simulink library "csc_src_slant_range_covariance_lib"  (R2015b)
settings: Solver=VariableStepAuto  StartTime=0.0  StopTime=10.0  RelTol=1e-3
values from neighbouring files (symbols this model uses):
  mnc_dtheta_filter_coeffs = [fir1(mnc_dtheta_filter_order(1),mnc_dtheta_filter_freq(1));,                               fir1(mnc_dtheta_filter_order(2),mnc_dtheta_filter_freq(2))]    [csc_mnc_measurement_noise_covariance_init.m]
  mnc_dtheta_filter_order = [1      1]    [csc_mnc_measurement_noise_covariance_init.m]
  mnc_meas_noise_alt = 8000.0    (= 8000)    [csc_mnc_measurement_noise_covariance_init.m]
  mnc_meas_noise_alt_gain = [0.2    0.2     1000   1000]    [csc_mnc_measurement_noise_covariance_init.m]
  mnc_meas_noise_angle_exp = [10     10]    [csc_mnc_measurement_noise_covariance_init.m]
  mnc_meas_noise_angle_gain = [1.0    1.0]    [csc_mnc_measurement_noise_covariance_init.m]
  mnc_meas_noise_angle_high = [90.0   20.0]    [csc_mnc_measurement_noise_covariance_init.m]
  mnc_meas_noise_angle_low = [10.0   10.0]    [csc_mnc_measurement_noise_covariance_init.m]
  mnc_meas_noise_angle_terminal = [10.0   10.0]    [csc_mnc_measurement_noise_covariance_init.m]
  mnc_meas_noise_dtheta = [4.0    4.0]    [csc_mnc_measurement_noise_covariance_init.m]
  mnc_meas_noise_dtheta_exp = [11     11]    [csc_mnc_measurement_noise_covariance_init.m]
  mnc_meas_noise_dtheta_gain = [0.0    0.0]    [csc_mnc_measurement_noise_covariance_init.m]
  mnc_nadir_cant_angle = [0.0   45.0]    [csc_mnc_measurement_noise_covariance_init.m]
  mnc_noise_switch_alt = [2000  2000]    [csc_mnc_measurement_noise_covariance_init.m]
  mnc_noise_terminal_alt = [ 100   100]    [csc_mnc_measurement_noise_covariance_init.m]
  mnc_R_lower_limit_alt = [0.0001 0.0001  10     10]    [csc_mnc_measurement_noise_covariance_init.m]
  mnc_R_lower_limit_angle = [0.0001 0.001]    [csc_mnc_measurement_noise_covariance_init.m]
  mnc_R_lower_limit_dtheta = [0.0001 0.0001]    [csc_mnc_measurement_noise_covariance_init.m]
libraries: simulink x8, util_info_lib x2
settings Model: Creator=Mark Agbayani  LastModifiedBy=Mark Agbayani

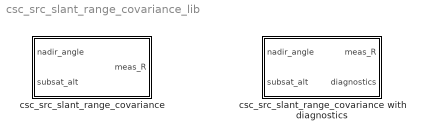
== system csc_src_slant_range_covariance_lib ==
  csc_src_slant_range_covariance : Subsystem  mask{i=0}
      mask prompts: i "Lidar Number"
  csc_src_slant_range_covariance with diagnostics : Subsystem  mask{i=0}
      mask prompts: i "Lidar Number"

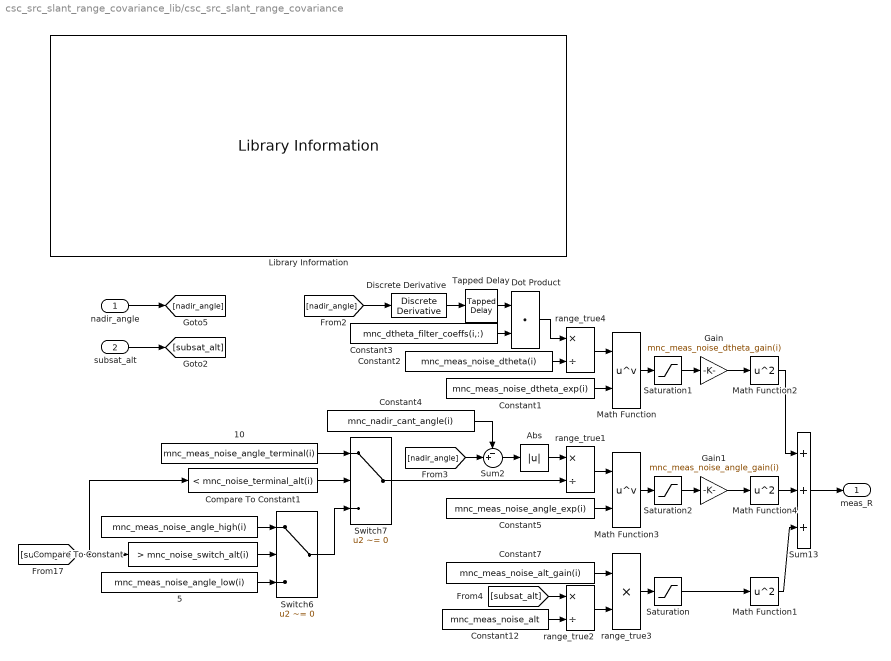
== system csc_src_slant_range_covariance_lib/csc_src_slant_range_covariance ==
  nadir_angle : Inport
  subsat_alt : Inport  Port=2
  "      " : Constant  Value=mnc_meas_noise_angle_high(i)
  "      10" : Constant  Value=mnc_meas_noise_angle_terminal(i)
  "      5" : Constant  Value=mnc_meas_noise_angle_low(i)
  Abs : Abs
  Compare To Constant : simulink/Logic and Bit Operations/Compare To Constant  relop=>  const=mnc_noise_switch_alt(i)  OutDataTypeStr=boolean
  Compare To Constant1 : simulink/Logic and Bit Operations/Compare To Constant  relop=<  const=mnc_noise_terminal_alt(i)  OutDataTypeStr=boolean
  Constant1 : Constant  Value=mnc_meas_noise_dtheta_exp(i)
  Constant12 : Constant  Value=mnc_meas_noise_alt
  Constant2 : Constant  Value=mnc_meas_noise_dtheta(i)
  Constant3 : Constant  Value=mnc_dtheta_filter_coeffs(i,:)
  Constant4 : Constant  Value=mnc_nadir_cant_angle(i)
  Constant5 : Constant  Value=mnc_meas_noise_angle_exp(i)
  Constant7 : Constant  Value=mnc_meas_noise_alt_gain(i)
  Discrete Derivative : simulink/Discrete/Discrete Derivative  gainval=1.0  ICPrevScaledInput=0.0  InputProcessing=Inherited  OutMin=[]  OutMax=[]  OutDataType=fixdt(1, 16)  OutScaling=2^-10  DoSatur=off
  Dot Product : DotProduct  InputSameDT=on  OutDataTypeStr=Inherit: Inherit via internal rule
  Gain : Gain  Gain=mnc_meas_noise_dtheta_gain(i)
  Gain1 : Gain  Gain=mnc_meas_noise_angle_gain(i)
  Library Information : util_info_lib/Library Information  owner='NONE'
  Math Function : Math  Operator=pow  SaturateOnIntegerOverflow=on
  Math Function1 : Math  Operator=square  SaturateOnIntegerOverflow=on
  Math Function2 : Math  Operator=square  SaturateOnIntegerOverflow=on
  Math Function3 : Math  Operator=pow  SaturateOnIntegerOverflow=on
  Math Function4 : Math  Operator=square  SaturateOnIntegerOverflow=on
  Saturation : Saturate  UpperLimit=1e20  LowerLimit=mnc_R_lower_limit_alt(i)
  Saturation1 : Saturate  UpperLimit=1e20  LowerLimit=mnc_R_lower_limit_dtheta(i)
  Saturation2 : Saturate  UpperLimit=1e20  LowerLimit=mnc_R_lower_limit_angle(i)
  Sum13 : Sum  Inputs=+++
  Sum2 : Sum  Inputs=-+|  AccumDataTypeStr=double
  Switch6 : Switch  Criteria=u2 ~= 0
  Switch7 : Switch  Criteria=u2 ~= 0
  Tapped Delay : simulink/Discrete/Tapped Delay  vinit=0.0  samptime=-1  NumDelays=mnc_dtheta_filter_order(i)  DelayOrder=Oldest  includeCurrent=on
  range_true1 : Product  Inputs=*/  RndMeth=Zero
  range_true2 : Product  Inputs=*/  RndMeth=Zero
  range_true3 : Product  RndMeth=Zero
  range_true4 : Product  Inputs=*/  RndMeth=Zero
  meas_R : Outport
  wires:
  nadir_angle/1 -> [nadir_angle]
  subsat_alt/1 -> [subsat_alt]
  Dot Product/1 -> range_true4/1
  Discrete Derivative/1 -> Tapped Delay/1
  Gain/1 -> Math Function2/1
  Gain1/1 -> Math Function4/1
  Constant5/1 -> Math Function3/2
  [nadir_angle] -> Discrete Derivative/1
  Switch7/1 -> range_true1/2
  Constant1/1 -> Math Function/2
  range_true1/1 -> Math Function3/1
  Math Function3/1 -> Saturation2/1
  Saturation2/1 -> Gain1/1
  Constant3/1 -> Dot Product/2
  Tapped Delay/1 -> Dot Product/1
  Math Function2/1 -> Sum13/1
  Constant2/1 -> range_true4/2
  range_true4/1 -> Math Function/1
  Math Function/1 -> Saturation1/1
  Saturation1/1 -> Gain/1
  Switch6/1 -> Switch7/3
  "      "/1 -> Switch6/1
  "      5"/1 -> Switch6/3
  Compare To Constant/1 -> Switch6/2
  [subsat_alt] -> Compare To Constant1/1, Compare To Constant/1
  "      10"/1 -> Switch7/1
  Compare To Constant1/1 -> Switch7/2
  Math Function4/1 -> Sum13/2
  range_true2/1 -> range_true3/2
  Constant7/1 -> range_true3/1
  range_true3/1 -> Saturation/1
  [subsat_alt] -> range_true2/1
  Constant12/1 -> range_true2/2
  Math Function1/1 -> Sum13/3
  Saturation/1 -> Math Function1/1
  Sum13/1 -> meas_R/1
  Constant4/1 -> Sum2/1
  Sum2/1 -> Abs/1
  [nadir_angle] -> Sum2/2
  Abs/1 -> range_true1/1

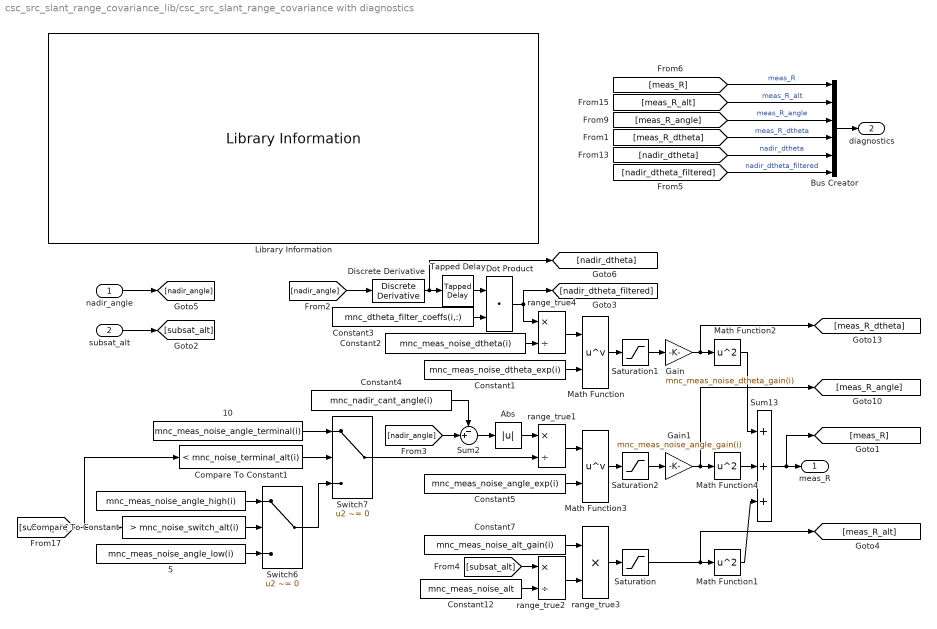
== system csc_src_slant_range_covariance_lib/csc_src_slant_range_covariance with diagnostics ==
  nadir_angle : Inport
  subsat_alt : Inport  Port=2
  "      " : Constant  Value=mnc_meas_noise_angle_high(i)
  "      10" : Constant  Value=mnc_meas_noise_angle_terminal(i)
  "      5" : Constant  Value=mnc_meas_noise_angle_low(i)
  Abs : Abs
  Bus Creator : BusCreator  Inputs=6
  Compare To Constant : simulink/Logic and Bit Operations/Compare To Constant  relop=>  const=mnc_noise_switch_alt(i)  OutDataTypeStr=boolean
  Compare To Constant1 : simulink/Logic and Bit Operations/Compare To Constant  relop=<  const=mnc_noise_terminal_alt(i)  OutDataTypeStr=boolean
  Constant1 : Constant  Value=mnc_meas_noise_dtheta_exp(i)
  Constant12 : Constant  Value=mnc_meas_noise_alt
  Constant2 : Constant  Value=mnc_meas_noise_dtheta(i)
  Constant3 : Constant  Value=mnc_dtheta_filter_coeffs(i,:)
  Constant4 : Constant  Value=mnc_nadir_cant_angle(i)
  Constant5 : Constant  Value=mnc_meas_noise_angle_exp(i)
  Constant7 : Constant  Value=mnc_meas_noise_alt_gain(i)
  Discrete Derivative : simulink/Discrete/Discrete Derivative  gainval=1.0  ICPrevScaledInput=0.0  InputProcessing=Inherited  OutMin=[]  OutMax=[]  OutDataType=fixdt(1, 16)  OutScaling=2^-10  DoSatur=off
  Dot Product : DotProduct  InputSameDT=on  OutDataTypeStr=Inherit: Inherit via internal rule
  Gain : Gain  Gain=mnc_meas_noise_dtheta_gain(i)
  Gain1 : Gain  Gain=mnc_meas_noise_angle_gain(i)
  Library Information : util_info_lib/Library Information  owner='NONE'
  Math Function : Math  Operator=pow  SaturateOnIntegerOverflow=on
  Math Function1 : Math  Operator=square  SaturateOnIntegerOverflow=on
  Math Function2 : Math  Operator=square  SaturateOnIntegerOverflow=on
  Math Function3 : Math  Operator=pow  SaturateOnIntegerOverflow=on
  Math Function4 : Math  Operator=square  SaturateOnIntegerOverflow=on
  Saturation : Saturate  UpperLimit=1e20  LowerLimit=mnc_R_lower_limit_alt(i)
  Saturation1 : Saturate  UpperLimit=1e20  LowerLimit=mnc_R_lower_limit_dtheta(i)
  Saturation2 : Saturate  UpperLimit=1e20  LowerLimit=mnc_R_lower_limit_angle(i)
  Sum13 : Sum  Inputs=+++
  Sum2 : Sum  Inputs=-+|  AccumDataTypeStr=double
  Switch6 : Switch  Criteria=u2 ~= 0
  Switch7 : Switch  Criteria=u2 ~= 0
  Tapped Delay : simulink/Discrete/Tapped Delay  vinit=0.0  samptime=-1  NumDelays=mnc_dtheta_filter_order(i)  DelayOrder=Oldest  includeCurrent=on
  range_true1 : Product  Inputs=*/  RndMeth=Zero
  range_true2 : Product  Inputs=*/  RndMeth=Zero
  range_true3 : Product  RndMeth=Zero
  range_true4 : Product  Inputs=*/  RndMeth=Zero
  meas_R : Outport
  diagnostics : Outport  Port=2
  wires:
  Constant4/1 -> Sum2/1
  Sum2/1 -> Abs/1
  [nadir_dtheta_filtered] -> Bus Creator/6  "nadir_dtheta_filtered"
  Bus Creator/1 -> diagnostics/1
  [meas_R] -> Bus Creator/1  "meas_R"
  [meas_R_alt] -> Bus Creator/2  "meas_R_alt"
  [nadir_dtheta] -> Bus Creator/5  "nadir_dtheta"
  [meas_R_angle] -> Bus Creator/3  "meas_R_angle"
  [meas_R_dtheta] -> Bus Creator/4  "meas_R_dtheta"
  nadir_angle/1 -> [nadir_angle]
  subsat_alt/1 -> [subsat_alt]
  [nadir_angle] -> Sum2/2
  Dot Product/1 -> range_true4/1, [nadir_dtheta_filtered]
  Discrete Derivative/1 -> Tapped Delay/1, [nadir_dtheta]
  Gain/1 -> Math Function2/1, [meas_R_dtheta]
  Gain1/1 -> Math Function4/1, [meas_R_angle]
  Constant5/1 -> Math Function3/2
  [nadir_angle] -> Discrete Derivative/1
  Switch7/1 -> range_true1/2
  Constant1/1 -> Math Function/2
  range_true1/1 -> Math Function3/1
  Math Function3/1 -> Saturation2/1
  Saturation2/1 -> Gain1/1
  Constant3/1 -> Dot Product/2
  Tapped Delay/1 -> Dot Product/1
  Math Function2/1 -> Sum13/1
  Constant2/1 -> range_true4/2
  range_true4/1 -> Math Function/1
  Math Function/1 -> Saturation1/1
  Saturation1/1 -> Gain/1
  Switch6/1 -> Switch7/3
  "      "/1 -> Switch6/1
  "      5"/1 -> Switch6/3
  Compare To Constant/1 -> Switch6/2
  [subsat_alt] -> Compare To Constant1/1, Compare To Constant/1
  "      10"/1 -> Switch7/1
  Compare To Constant1/1 -> Switch7/2
  Math Function4/1 -> Sum13/2
  range_true2/1 -> range_true3/2
  Constant7/1 -> range_true3/1
  range_true3/1 -> Saturation/1
  [subsat_alt] -> range_true2/1
  Constant12/1 -> range_true2/2
  Math Function1/1 -> Sum13/3
  Saturation/1 -> Math Function1/1, [meas_R_alt]
  Sum13/1 -> meas_R/1, [meas_R]
  Abs/1 -> range_true1/1
